simulink model "RobustStateSpaceSim"  (R2020b)
settings: Solver=ode45  StartTime=0.0  StopTime=10  RelTol=1e-3
undefined symbols (not defined in the file or in its folder): daq, degs2rpm, drv, gbox, mech, mld, mot, rads2rpm, robust, rpm2rads, sens, state_space
libraries: simulink x1
settings Model: Creator=Utente  LastModifiedBy=Utente

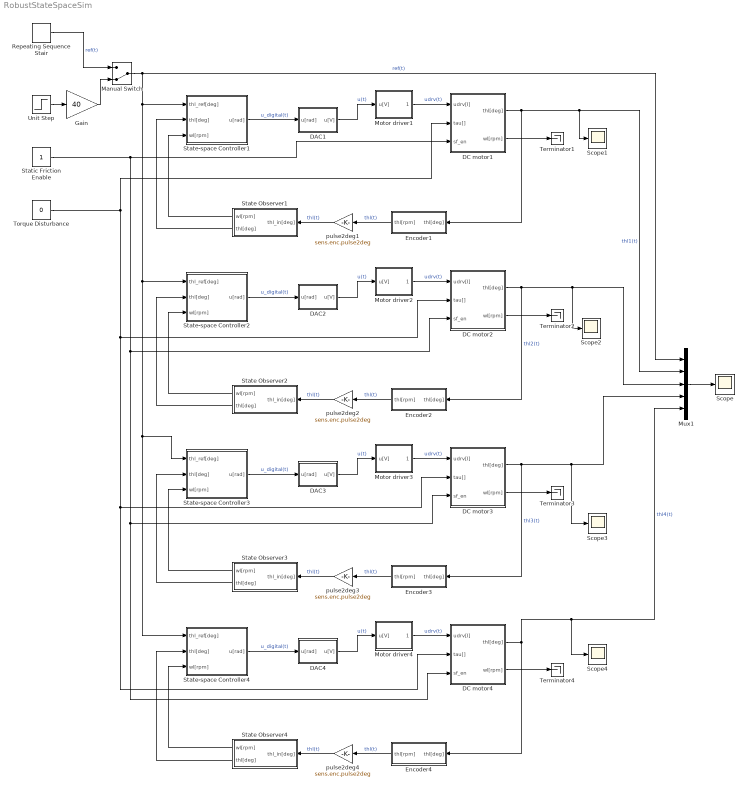
== system RobustStateSpaceSim ==
  DAC1 : Subsystem
  DAC2 : Subsystem
  DAC3 : Subsystem
  DAC4 : Subsystem
  DC motor1 : Subsystem
  DC motor2 : Subsystem
  DC motor3 : Subsystem
  DC motor4 : Subsystem
  Encoder1 : Subsystem
  Encoder2 : Subsystem
  Encoder3 : Subsystem
  Encoder4 : Subsystem
  Gain : Gain  Gain=40
  Manual Switch : ManualSwitch  CurrentSetting=0
  Motor driver1 : Subsystem
  Motor driver2 : Subsystem
  Motor driver3 : Subsystem
  Motor driver4 : Subsystem
  Mux1 : Mux  Inputs=5
  Repeating Sequence Stair : simulink/Sources/Repeating Sequence Stair  OutValues=[40 0 70 0 120 0].'  tsamp=2  OutMin=[]  OutMax=[]  OutDataTypeStr=double  OutputDataTypeScalingMode=double  OutDataType=fixdt(0,8)  ConRadixGroup=Best Precision: Vector-wise  OutScaling=2^-12
  Scope{,1..4} (5 alike) : Scope
  State Observer1 : Subsystem
  State Observer2 : Subsystem
  State Observer3 : Subsystem
  State Observer4 : Subsystem
  State-space Controller1 : Subsystem
  State-space Controller2 : Subsystem
  State-space Controller3 : Subsystem
  State-space Controller4 : Subsystem
  Static Friction Enable : Constant
  Terminator{1..4} (4 alike) : Terminator
  Torque Disturbance : Constant  Value=0
  Unit Step : Step  Time=0  SampleTime=0
  pulse2deg{1..4} (4 alike) : Gain  Gain=sens.enc.pulse2deg
  wires:
  State Observer4/2(thl[deg]) -> State-space Controller4/2(thl[deg])
  Motor driver3/1(udrv[I]) -> DC motor3/1(udrv[I])  "udrv(t)"
  State Observer4/1(wl[rpm]) -> State-space Controller4/3(wl[rpm])
  DC motor4/2(wl[rpm]) -> Terminator4/1
  DC motor3/1(thl[deg]) -> Scope3/1, Mux1/4, Encoder3/1(thl[deg])  "thl3(t)"
  DAC3/1(u[V]) -> Motor driver3/1(u[V])  "u(t)"
  State-space Controller3/1(u[rad]) -> DAC3/1(u[rad])  "u_digital(t)"
  Encoder4/1(thl[rpm]) -> pulse2deg4/1  "thl(t)"
  DC motor4/1(thl[deg]) -> Scope4/1, Mux1/5, Encoder4/1(thl[deg])  "thl4(t)"
  pulse2deg2/1 -> State Observer2/1(thl_in[deg])  "thl(t)"
  Encoder2/1(thl[rpm]) -> pulse2deg2/1  "thl(t)"
  Motor driver4/1(udrv[I]) -> DC motor4/1(udrv[I])  "udrv(t)"
  DC motor2/1(thl[deg]) -> Encoder2/1(thl[deg]), Scope2/1, Mux1/3  "thl2(t)"
  Motor driver2/1(udrv[I]) -> DC motor2/1(udrv[I])  "udrv(t)"
  DC motor3/2(wl[rpm]) -> Terminator3/1
  Manual Switch/1 -> State-space Controller3/1(thl_ref[deg]), State-space Controller4/1(thl_ref[deg]), State-space Controller2/1(thl_ref[deg]), State-space Controller1/1(thl_ref[deg]), Mux1/1  "ref(t)"
  DAC2/1(u[V]) -> Motor driver2/1(u[V])  "u(t)"
  State-space Controller2/1(u[rad]) -> DAC2/1(u[rad])  "u_digital(t)"
  State Observer1/1(wl[rpm]) -> State-space Controller1/3(wl[rpm])
  Encoder3/1(thl[rpm]) -> pulse2deg3/1  "thl(t)"
  State-space Controller1/1(u[rad]) -> DAC1/1(u[rad])  "u_digital(t)"
  pulse2deg1/1 -> State Observer1/1(thl_in[deg])  "thl(t)"
  State Observer3/1(wl[rpm]) -> State-space Controller3/3(wl[rpm])
  State Observer1/2(thl[deg]) -> State-space Controller1/2(thl[deg])
  DAC1/1(u[V]) -> Motor driver1/1(u[V])  "u(t)"
  DC motor2/2(wl[rpm]) -> Terminator2/1
  DC motor1/1(thl[deg]) -> Scope1/1, Mux1/2, Encoder1/1(thl[deg])  "thl1(t)"
  Encoder1/1(thl[rpm]) -> pulse2deg1/1  "thl(t)"
  DAC4/1(u[V]) -> Motor driver4/1(u[V])  "u(t)"
  State Observer2/1(wl[rpm]) -> State-space Controller2/3(wl[rpm])
  Motor driver1/1(udrv[I]) -> DC motor1/1(udrv[I])  "udrv(t)"
  State Observer3/2(thl[deg]) -> State-space Controller3/2(thl[deg])
  Torque Disturbance/1 -> DC motor3/2(tau[]), DC motor4/2(tau[]), DC motor2/2(tau[]), DC motor1/2(tau[])
  State-space Controller4/1(u[rad]) -> DAC4/1(u[rad])  "u_digital(t)"
  Static Friction Enable/1 -> DC motor1/3(sf_en), DC motor2/3(sf_en), DC motor3/3(sf_en), DC motor4/3(sf_en)
  pulse2deg4/1 -> State Observer4/1(thl_in[deg])  "thl(t)"
  State Observer2/2(thl[deg]) -> State-space Controller2/2(thl[deg])
  pulse2deg3/1 -> State Observer3/1(thl_in[deg])  "thl(t)"
  DC motor1/2(wl[rpm]) -> Terminator1/1
  Mux1/1 -> Scope/1
  Repeating Sequence Stair/1 -> Manual Switch/1  "ref(t)"
  Unit Step/1 -> Gain/1
  Gain/1 -> Manual Switch/2

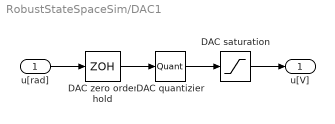
== system RobustStateSpaceSim/DAC1 ==
  u[rad] : Inport
  DAC quantizier : Quantizer  QuantizationInterval=daq.dac.q
  DAC saturation : Saturate  UpperLimit=daq.dac.vdd  LowerLimit=daq.dac.vss
  DAC zero order hold : ZeroOrderHold  SampleTime=daq.dac.T_s
  u[V] : Outport
  wires:
  DAC quantizier/1 -> DAC saturation/1
  DAC zero order hold/1 -> DAC quantizier/1
  DAC saturation/1 -> u[V]/1
  u[rad]/1 -> DAC zero order hold/1

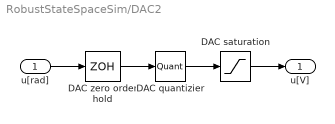
== system RobustStateSpaceSim/DAC2 ==
  u[rad] : Inport
  DAC quantizier : Quantizer  QuantizationInterval=daq.dac.q
  DAC saturation : Saturate  UpperLimit=daq.dac.vdd  LowerLimit=daq.dac.vss
  DAC zero order hold : ZeroOrderHold  SampleTime=daq.dac.T_s
  u[V] : Outport
  wires:
  DAC quantizier/1 -> DAC saturation/1
  DAC zero order hold/1 -> DAC quantizier/1
  DAC saturation/1 -> u[V]/1
  u[rad]/1 -> DAC zero order hold/1

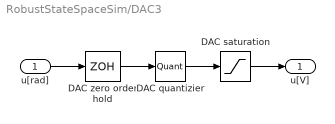
== system RobustStateSpaceSim/DAC3 ==
  u[rad] : Inport
  DAC quantizier : Quantizer  QuantizationInterval=daq.dac.q
  DAC saturation : Saturate  UpperLimit=daq.dac.vdd  LowerLimit=daq.dac.vss
  DAC zero order hold : ZeroOrderHold  SampleTime=daq.dac.T_s
  u[V] : Outport
  wires:
  DAC quantizier/1 -> DAC saturation/1
  DAC zero order hold/1 -> DAC quantizier/1
  DAC saturation/1 -> u[V]/1
  u[rad]/1 -> DAC zero order hold/1

== system RobustStateSpaceSim/DAC4 ==
  u[rad] : Inport
  DAC quantizier : Quantizer  QuantizationInterval=daq.dac.q
  DAC saturation : Saturate  UpperLimit=daq.dac.vdd  LowerLimit=daq.dac.vss
  DAC zero order hold : ZeroOrderHold  SampleTime=daq.dac.T_s
  u[V] : Outport
  wires:
  DAC quantizier/1 -> DAC saturation/1
  DAC zero order hold/1 -> DAC quantizier/1
  DAC saturation/1 -> u[V]/1
  u[rad]/1 -> DAC zero order hold/1

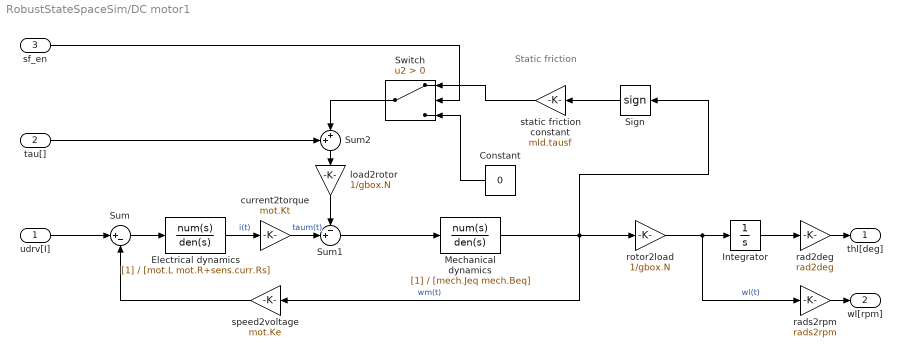
== system RobustStateSpaceSim/DC motor1 ==
  note: Static friction
  udrv[I] : Inport  Unit=V
  tau[] : Inport  Port=2  Unit=V
  sf_en : Inport  Port=3  Unit=V
  Constant : Constant  Value=0
  Electrical dynamics : TransferFcn  Denominator=[mot.L mot.R+sens.curr.Rs]
  Integrator : Integrator
  Mechanical dynamics : TransferFcn  Denominator=[mech.Jeq mech.Beq]
  Sign : Signum  ZeroCross=off
  Sum : Sum  Inputs=|+-
  Sum1 : Sum  Inputs=-+|
  Sum2 : Sum  Inputs=++|
  Switch : Switch  Criteria=u2 > Threshold
  current2torque : Gain  Gain=mot.Kt
  load2rotor : Gain  Gain=1/gbox.N
  rad2deg : Gain  Gain=rad2deg
  rads2rpm : Gain  Gain=rads2rpm
  rotor2load : Gain  Gain=1/gbox.N
  speed2voltage : Gain  Gain=mot.Ke
  static friction constant : Gain  Gain=mld.tausf
  thl[deg] : Outport  Unit=deg
  wl[rpm] : Outport  Port=2  Unit=rpm
  wires:
  load2rotor/1 -> Sum1/1
  Mechanical dynamics/1 -> Sign/1, rotor2load/1, speed2voltage/1  "wm(t)"
  Sign/1 -> static friction constant/1
  current2torque/1 -> Sum1/2  "taum(t)"
  Sum1/1 -> Mechanical dynamics/1
  speed2voltage/1 -> Sum/2
  rotor2load/1 -> rads2rpm/1, Integrator/1  "wl(t)"
  Electrical dynamics/1 -> current2torque/1  "i(t)"
  Integrator/1 -> rad2deg/1
  Sum/1 -> Electrical dynamics/1
  rads2rpm/1 -> wl[rpm]/1
  rad2deg/1 -> thl[deg]/1
  udrv[I]/1 -> Sum/1
  Sum2/1 -> load2rotor/1
  tau[]/1 -> Sum2/1
  Switch/1 -> Sum2/2
  static friction constant/1 -> Switch/1
  Constant/1 -> Switch/3
  sf_en/1 -> Switch/2

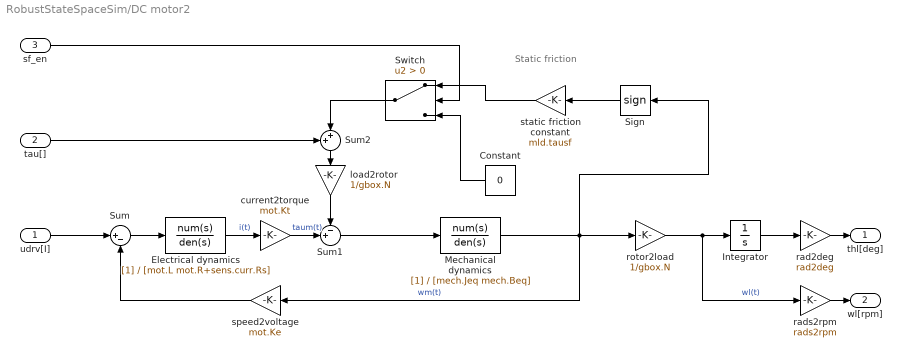
== system RobustStateSpaceSim/DC motor2 ==
  note: Static friction
  udrv[I] : Inport  Unit=V
  tau[] : Inport  Port=2  Unit=V
  sf_en : Inport  Port=3  Unit=V
  Constant : Constant  Value=0
  Electrical dynamics : TransferFcn  Denominator=[mot.L mot.R+sens.curr.Rs]
  Integrator : Integrator
  Mechanical dynamics : TransferFcn  Denominator=[mech.Jeq mech.Beq]
  Sign : Signum  ZeroCross=off
  Sum : Sum  Inputs=|+-
  Sum1 : Sum  Inputs=-+|
  Sum2 : Sum  Inputs=++|
  Switch : Switch  Criteria=u2 > Threshold
  current2torque : Gain  Gain=mot.Kt
  load2rotor : Gain  Gain=1/gbox.N
  rad2deg : Gain  Gain=rad2deg
  rads2rpm : Gain  Gain=rads2rpm
  rotor2load : Gain  Gain=1/gbox.N
  speed2voltage : Gain  Gain=mot.Ke
  static friction constant : Gain  Gain=mld.tausf
  thl[deg] : Outport  Unit=deg
  wl[rpm] : Outport  Port=2  Unit=rpm
  wires:
  load2rotor/1 -> Sum1/1
  Mechanical dynamics/1 -> Sign/1, rotor2load/1, speed2voltage/1  "wm(t)"
  Sign/1 -> static friction constant/1
  current2torque/1 -> Sum1/2  "taum(t)"
  Sum1/1 -> Mechanical dynamics/1
  speed2voltage/1 -> Sum/2
  rotor2load/1 -> rads2rpm/1, Integrator/1  "wl(t)"
  Electrical dynamics/1 -> current2torque/1  "i(t)"
  Integrator/1 -> rad2deg/1
  Sum/1 -> Electrical dynamics/1
  rads2rpm/1 -> wl[rpm]/1
  rad2deg/1 -> thl[deg]/1
  udrv[I]/1 -> Sum/1
  Sum2/1 -> load2rotor/1
  tau[]/1 -> Sum2/1
  Switch/1 -> Sum2/2
  static friction constant/1 -> Switch/1
  Constant/1 -> Switch/3
  sf_en/1 -> Switch/2

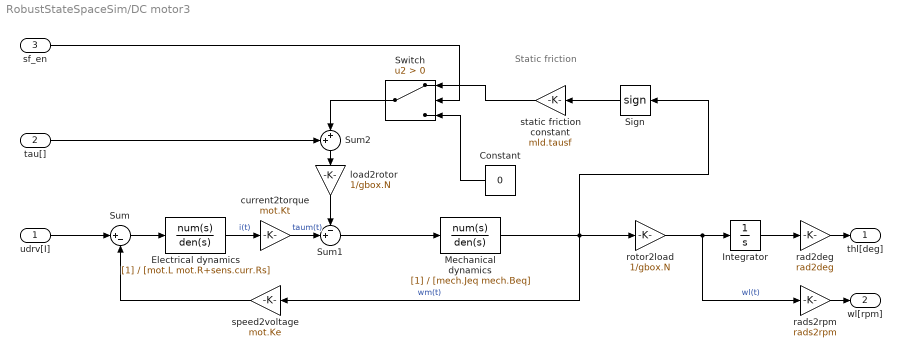
== system RobustStateSpaceSim/DC motor3 ==
  note: Static friction
  udrv[I] : Inport  Unit=V
  tau[] : Inport  Port=2  Unit=V
  sf_en : Inport  Port=3  Unit=V
  Constant : Constant  Value=0
  Electrical dynamics : TransferFcn  Denominator=[mot.L mot.R+sens.curr.Rs]
  Integrator : Integrator
  Mechanical dynamics : TransferFcn  Denominator=[mech.Jeq mech.Beq]
  Sign : Signum  ZeroCross=off
  Sum : Sum  Inputs=|+-
  Sum1 : Sum  Inputs=-+|
  Sum2 : Sum  Inputs=++|
  Switch : Switch  Criteria=u2 > Threshold
  current2torque : Gain  Gain=mot.Kt
  load2rotor : Gain  Gain=1/gbox.N
  rad2deg : Gain  Gain=rad2deg
  rads2rpm : Gain  Gain=rads2rpm
  rotor2load : Gain  Gain=1/gbox.N
  speed2voltage : Gain  Gain=mot.Ke
  static friction constant : Gain  Gain=mld.tausf
  thl[deg] : Outport  Unit=deg
  wl[rpm] : Outport  Port=2  Unit=rpm
  wires:
  load2rotor/1 -> Sum1/1
  Mechanical dynamics/1 -> Sign/1, rotor2load/1, speed2voltage/1  "wm(t)"
  Sign/1 -> static friction constant/1
  current2torque/1 -> Sum1/2  "taum(t)"
  Sum1/1 -> Mechanical dynamics/1
  speed2voltage/1 -> Sum/2
  rotor2load/1 -> rads2rpm/1, Integrator/1  "wl(t)"
  Electrical dynamics/1 -> current2torque/1  "i(t)"
  Integrator/1 -> rad2deg/1
  Sum/1 -> Electrical dynamics/1
  rads2rpm/1 -> wl[rpm]/1
  rad2deg/1 -> thl[deg]/1
  udrv[I]/1 -> Sum/1
  Sum2/1 -> load2rotor/1
  tau[]/1 -> Sum2/1
  Switch/1 -> Sum2/2
  static friction constant/1 -> Switch/1
  Constant/1 -> Switch/3
  sf_en/1 -> Switch/2

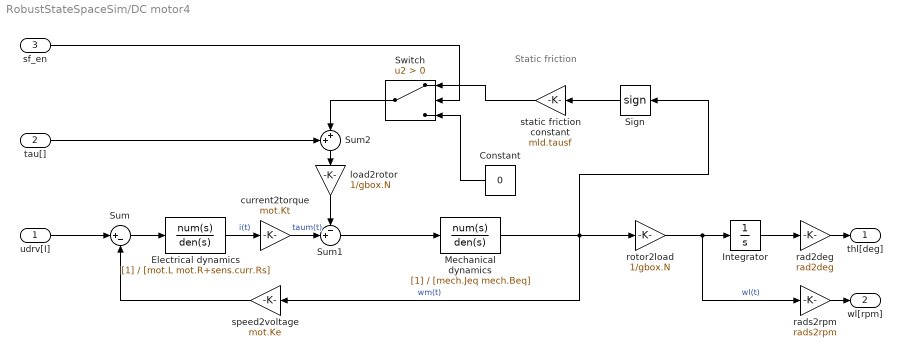
== system RobustStateSpaceSim/DC motor4 ==
  note: Static friction
  udrv[I] : Inport  Unit=V
  tau[] : Inport  Port=2  Unit=V
  sf_en : Inport  Port=3  Unit=V
  Constant : Constant  Value=0
  Electrical dynamics : TransferFcn  Denominator=[mot.L mot.R+sens.curr.Rs]
  Integrator : Integrator
  Mechanical dynamics : TransferFcn  Denominator=[mech.Jeq mech.Beq]
  Sign : Signum  ZeroCross=off
  Sum : Sum  Inputs=|+-
  Sum1 : Sum  Inputs=-+|
  Sum2 : Sum  Inputs=++|
  Switch : Switch  Criteria=u2 > Threshold
  current2torque : Gain  Gain=mot.Kt
  load2rotor : Gain  Gain=1/gbox.N
  rad2deg : Gain  Gain=rad2deg
  rads2rpm : Gain  Gain=rads2rpm
  rotor2load : Gain  Gain=1/gbox.N
  speed2voltage : Gain  Gain=mot.Ke
  static friction constant : Gain  Gain=mld.tausf
  thl[deg] : Outport  Unit=deg
  wl[rpm] : Outport  Port=2  Unit=rpm
  wires:
  load2rotor/1 -> Sum1/1
  Mechanical dynamics/1 -> Sign/1, rotor2load/1, speed2voltage/1  "wm(t)"
  Sign/1 -> static friction constant/1
  current2torque/1 -> Sum1/2  "taum(t)"
  Sum1/1 -> Mechanical dynamics/1
  speed2voltage/1 -> Sum/2
  rotor2load/1 -> rads2rpm/1, Integrator/1  "wl(t)"
  Electrical dynamics/1 -> current2torque/1  "i(t)"
  Integrator/1 -> rad2deg/1
  Sum/1 -> Electrical dynamics/1
  rads2rpm/1 -> wl[rpm]/1
  rad2deg/1 -> thl[deg]/1
  udrv[I]/1 -> Sum/1
  Sum2/1 -> load2rotor/1
  tau[]/1 -> Sum2/1
  Switch/1 -> Sum2/2
  static friction constant/1 -> Switch/1
  Constant/1 -> Switch/3
  sf_en/1 -> Switch/2

== system RobustStateSpaceSim/Encoder1 ==
  thl[deg] : Inport
  Encoder quantization : Quantizer  QuantizationInterval=sens.enc.q
  Encoder sampling : ZeroOrderHold  SampleTime=sens.enc.T_s
  deg2pulse : Gain  Gain=sens.enc.deg2pulse
  thl[rpm] : Outport
  wires:
  Encoder quantization/1 -> deg2pulse/1
  deg2pulse/1 -> thl[rpm]/1
  Encoder sampling/1 -> Encoder quantization/1
  thl[deg]/1 -> Encoder sampling/1

== system RobustStateSpaceSim/Encoder2 ==
  thl[deg] : Inport
  Encoder quantization : Quantizer  QuantizationInterval=sens.enc.q
  Encoder sampling : ZeroOrderHold  SampleTime=sens.enc.T_s
  deg2pulse : Gain  Gain=sens.enc.deg2pulse
  thl[rpm] : Outport
  wires:
  Encoder quantization/1 -> deg2pulse/1
  deg2pulse/1 -> thl[rpm]/1
  Encoder sampling/1 -> Encoder quantization/1
  thl[deg]/1 -> Encoder sampling/1

== system RobustStateSpaceSim/Encoder3 ==
  thl[deg] : Inport
  Encoder quantization : Quantizer  QuantizationInterval=sens.enc.q
  Encoder sampling : ZeroOrderHold  SampleTime=sens.enc.T_s
  deg2pulse : Gain  Gain=sens.enc.deg2pulse
  thl[rpm] : Outport
  wires:
  Encoder quantization/1 -> deg2pulse/1
  deg2pulse/1 -> thl[rpm]/1
  Encoder sampling/1 -> Encoder quantization/1
  thl[deg]/1 -> Encoder sampling/1

== system RobustStateSpaceSim/Encoder4 ==
  thl[deg] : Inport
  Encoder quantization : Quantizer  QuantizationInterval=sens.enc.q
  Encoder sampling : ZeroOrderHold  SampleTime=sens.enc.T_s
  deg2pulse : Gain  Gain=sens.enc.deg2pulse
  thl[rpm] : Outport
  wires:
  Encoder quantization/1 -> deg2pulse/1
  deg2pulse/1 -> thl[rpm]/1
  Encoder sampling/1 -> Encoder quantization/1
  thl[deg]/1 -> Encoder sampling/1

== system RobustStateSpaceSim/Motor driver1 ==
  u[V] : Inport
  Driver dynamics : TransferFcn  Numerator=[drv.dcgain]  Denominator=[drv.Tc 1]
  Driver saturation : Saturate  UpperLimit=drv.vp  LowerLimit=drv.vm
  udrv[I] : Outport
  wires:
  Driver saturation/1 -> udrv[I]/1
  Driver dynamics/1 -> Driver saturation/1
  u[V]/1 -> Driver dynamics/1

== system RobustStateSpaceSim/Motor driver2 ==
  u[V] : Inport
  Driver dynamics : TransferFcn  Numerator=[drv.dcgain]  Denominator=[drv.Tc 1]
  Driver saturation : Saturate  UpperLimit=drv.vp  LowerLimit=drv.vm
  udrv[I] : Outport
  wires:
  Driver saturation/1 -> udrv[I]/1
  Driver dynamics/1 -> Driver saturation/1
  u[V]/1 -> Driver dynamics/1

== system RobustStateSpaceSim/Motor driver3 ==
  u[V] : Inport
  Driver dynamics : TransferFcn  Numerator=[drv.dcgain]  Denominator=[drv.Tc 1]
  Driver saturation : Saturate  UpperLimit=drv.vp  LowerLimit=drv.vm
  udrv[I] : Outport
  wires:
  Driver saturation/1 -> udrv[I]/1
  Driver dynamics/1 -> Driver saturation/1
  u[V]/1 -> Driver dynamics/1

== system RobustStateSpaceSim/Motor driver4 ==
  u[V] : Inport
  Driver dynamics : TransferFcn  Numerator=[drv.dcgain]  Denominator=[drv.Tc 1]
  Driver saturation : Saturate  UpperLimit=drv.vp  LowerLimit=drv.vm
  udrv[I] : Outport
  wires:
  Driver saturation/1 -> udrv[I]/1
  Driver dynamics/1 -> Driver saturation/1
  u[V]/1 -> Driver dynamics/1

== system RobustStateSpaceSim/State Observer1 ==
  thl_in[deg] : Inport
  Gain1 : Gain  Gain=degs2rpm
  Transfer Fcn : TransferFcn  Numerator=[state_space.obs.wc^2 0]  Denominator=[1 2*state_space.obs.delta*state_space.obs.wc state_space.obs.wc^2]
  wl[rpm] : Outport
  thl[deg] : Outport  Port=2
  wires:
  Transfer Fcn/1 -> Gain1/1
  thl_in[deg]/1 -> thl[deg]/1, Transfer Fcn/1
  Gain1/1 -> wl[rpm]/1

== system RobustStateSpaceSim/State Observer2 ==
  thl_in[deg] : Inport
  Gain1 : Gain  Gain=degs2rpm
  Transfer Fcn : TransferFcn  Numerator=[state_space.obs.wc^2 0]  Denominator=[1 2*state_space.obs.delta*state_space.obs.wc state_space.obs.wc^2]
  wl[rpm] : Outport
  thl[deg] : Outport  Port=2
  wires:
  Transfer Fcn/1 -> Gain1/1
  thl_in[deg]/1 -> thl[deg]/1, Transfer Fcn/1
  Gain1/1 -> wl[rpm]/1

== system RobustStateSpaceSim/State Observer3 ==
  thl_in[deg] : Inport
  Gain1 : Gain  Gain=degs2rpm
  Transfer Fcn : TransferFcn  Numerator=[state_space.obs.wc^2 0]  Denominator=[1 2*state_space.obs.delta*state_space.obs.wc state_space.obs.wc^2]
  wl[rpm] : Outport
  thl[deg] : Outport  Port=2
  wires:
  Transfer Fcn/1 -> Gain1/1
  thl_in[deg]/1 -> thl[deg]/1, Transfer Fcn/1
  Gain1/1 -> wl[rpm]/1

== system RobustStateSpaceSim/State Observer4 ==
  thl_in[deg] : Inport
  Gain1 : Gain  Gain=degs2rpm
  Transfer Fcn : TransferFcn  Numerator=[state_space.obs.wc^2 0]  Denominator=[1 2*state_space.obs.delta*state_space.obs.wc state_space.obs.wc^2]
  wl[rpm] : Outport
  thl[deg] : Outport  Port=2
  wires:
  Transfer Fcn/1 -> Gain1/1
  thl_in[deg]/1 -> thl[deg]/1, Transfer Fcn/1
  Gain1/1 -> wl[rpm]/1

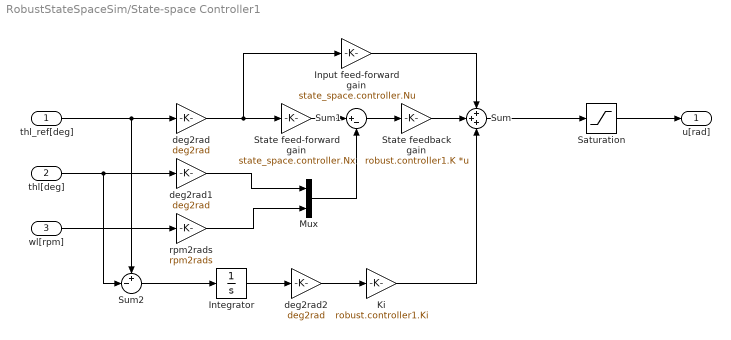
== system RobustStateSpaceSim/State-space Controller1 ==
  thl_ref[deg] : Inport
  thl[deg] : Inport  Port=2
  wl[rpm] : Inport  Port=3
  Input feed-forward gain : Gain  Gain=state_space.controller.Nu
  Integrator : Integrator
  Ki : Gain  Gain=robust.controller1.Ki
  Mux : Mux  Inputs=2
  Saturation : Saturate  UpperLimit=daq.dac.vdd  LowerLimit=daq.dac.vss
  State feed-forward gain : Gain  Gain=state_space.controller.Nx
  State feedback gain : Gain  Gain=robust.controller1.K  Multiplication=Matrix(K*u)
  Sum : Sum  Inputs=+++
  Sum1 : Sum  Inputs=|+-
  Sum2 : Sum  Inputs=+-|
  deg2rad : Gain  Gain=deg2rad
  deg2rad1 : Gain  Gain=deg2rad
  deg2rad2 : Gain  Gain=deg2rad
  rpm2rads : Gain  Gain=rpm2rads
  u[rad] : Outport
  wires:
  rpm2rads/1 -> Mux/2
  Sum1/1 -> State feedback gain/1
  Mux/1 -> Sum1/2
  thl_ref[deg]/1 -> Sum2/1, deg2rad/1
  deg2rad/1 -> Input feed-forward gain/1, State feed-forward gain/1
  State feed-forward gain/1 -> Sum1/1
  deg2rad1/1 -> Mux/1
  Input feed-forward gain/1 -> Sum/1
  Saturation/1 -> u[rad]/1
  wl[rpm]/1 -> rpm2rads/1
  thl[deg]/1 -> Sum2/2, deg2rad1/1
  State feedback gain/1 -> Sum/2
  Sum/1 -> Saturation/1
  Sum2/1 -> Integrator/1
  Integrator/1 -> deg2rad2/1
  deg2rad2/1 -> Ki/1
  Ki/1 -> Sum/3

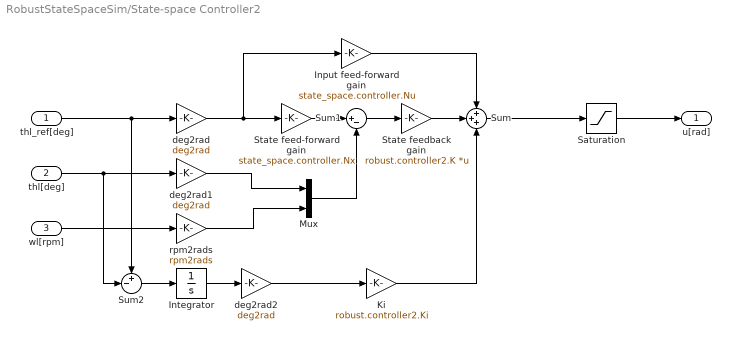
== system RobustStateSpaceSim/State-space Controller2 ==
  thl_ref[deg] : Inport
  thl[deg] : Inport  Port=2
  wl[rpm] : Inport  Port=3
  Input feed-forward gain : Gain  Gain=state_space.controller.Nu
  Integrator : Integrator
  Ki : Gain  Gain=robust.controller2.Ki
  Mux : Mux  Inputs=2
  Saturation : Saturate  UpperLimit=daq.dac.vdd  LowerLimit=daq.dac.vss
  State feed-forward gain : Gain  Gain=state_space.controller.Nx
  State feedback gain : Gain  Gain=robust.controller2.K  Multiplication=Matrix(K*u)
  Sum : Sum  Inputs=+++
  Sum1 : Sum  Inputs=|+-
  Sum2 : Sum  Inputs=+-|
  deg2rad : Gain  Gain=deg2rad
  deg2rad1 : Gain  Gain=deg2rad
  deg2rad2 : Gain  Gain=deg2rad
  rpm2rads : Gain  Gain=rpm2rads
  u[rad] : Outport
  wires:
  rpm2rads/1 -> Mux/2
  Sum1/1 -> State feedback gain/1
  Mux/1 -> Sum1/2
  thl_ref[deg]/1 -> Sum2/1, deg2rad/1
  deg2rad/1 -> Input feed-forward gain/1, State feed-forward gain/1
  State feed-forward gain/1 -> Sum1/1
  deg2rad1/1 -> Mux/1
  Input feed-forward gain/1 -> Sum/1
  Saturation/1 -> u[rad]/1
  wl[rpm]/1 -> rpm2rads/1
  thl[deg]/1 -> Sum2/2, deg2rad1/1
  State feedback gain/1 -> Sum/2
  Sum/1 -> Saturation/1
  Sum2/1 -> Integrator/1
  Integrator/1 -> deg2rad2/1
  deg2rad2/1 -> Ki/1
  Ki/1 -> Sum/3

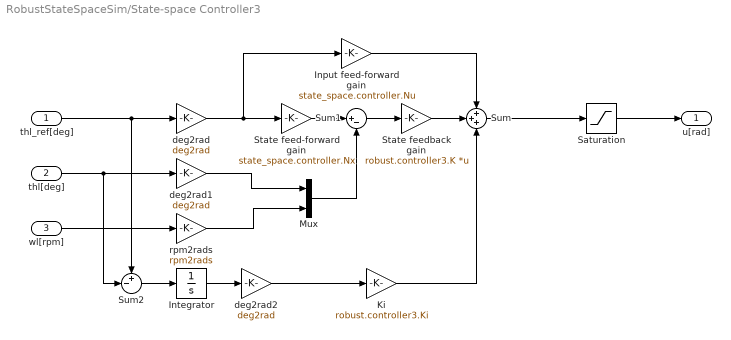
== system RobustStateSpaceSim/State-space Controller3 ==
  thl_ref[deg] : Inport
  thl[deg] : Inport  Port=2
  wl[rpm] : Inport  Port=3
  Input feed-forward gain : Gain  Gain=state_space.controller.Nu
  Integrator : Integrator
  Ki : Gain  Gain=robust.controller3.Ki
  Mux : Mux  Inputs=2
  Saturation : Saturate  UpperLimit=daq.dac.vdd  LowerLimit=daq.dac.vss
  State feed-forward gain : Gain  Gain=state_space.controller.Nx
  State feedback gain : Gain  Gain=robust.controller3.K  Multiplication=Matrix(K*u)
  Sum : Sum  Inputs=+++
  Sum1 : Sum  Inputs=|+-
  Sum2 : Sum  Inputs=+-|
  deg2rad : Gain  Gain=deg2rad
  deg2rad1 : Gain  Gain=deg2rad
  deg2rad2 : Gain  Gain=deg2rad
  rpm2rads : Gain  Gain=rpm2rads
  u[rad] : Outport
  wires:
  rpm2rads/1 -> Mux/2
  Sum1/1 -> State feedback gain/1
  Mux/1 -> Sum1/2
  thl_ref[deg]/1 -> Sum2/1, deg2rad/1
  deg2rad/1 -> Input feed-forward gain/1, State feed-forward gain/1
  State feed-forward gain/1 -> Sum1/1
  deg2rad1/1 -> Mux/1
  Input feed-forward gain/1 -> Sum/1
  Saturation/1 -> u[rad]/1
  wl[rpm]/1 -> rpm2rads/1
  thl[deg]/1 -> Sum2/2, deg2rad1/1
  State feedback gain/1 -> Sum/2
  Sum/1 -> Saturation/1
  Sum2/1 -> Integrator/1
  Integrator/1 -> deg2rad2/1
  deg2rad2/1 -> Ki/1
  Ki/1 -> Sum/3

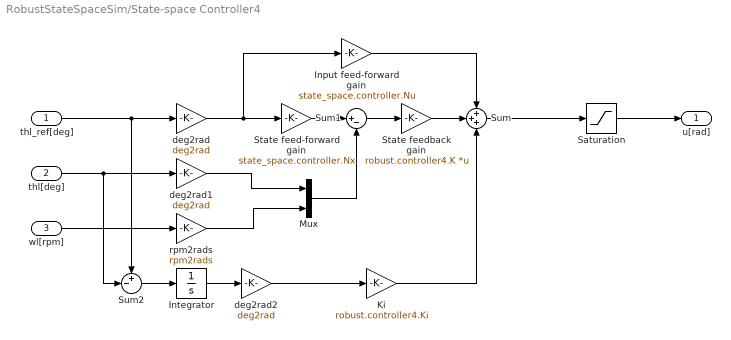
== system RobustStateSpaceSim/State-space Controller4 ==
  thl_ref[deg] : Inport
  thl[deg] : Inport  Port=2
  wl[rpm] : Inport  Port=3
  Input feed-forward gain : Gain  Gain=state_space.controller.Nu
  Integrator : Integrator
  Ki : Gain  Gain=robust.controller4.Ki
  Mux : Mux  Inputs=2
  Saturation : Saturate  UpperLimit=daq.dac.vdd  LowerLimit=daq.dac.vss
  State feed-forward gain : Gain  Gain=state_space.controller.Nx
  State feedback gain : Gain  Gain=robust.controller4.K  Multiplication=Matrix(K*u)
  Sum : Sum  Inputs=+++
  Sum1 : Sum  Inputs=|+-
  Sum2 : Sum  Inputs=+-|
  deg2rad : Gain  Gain=deg2rad
  deg2rad1 : Gain  Gain=deg2rad
  deg2rad2 : Gain  Gain=deg2rad
  rpm2rads : Gain  Gain=rpm2rads
  u[rad] : Outport
  wires:
  rpm2rads/1 -> Mux/2
  Sum1/1 -> State feedback gain/1
  Mux/1 -> Sum1/2
  thl_ref[deg]/1 -> Sum2/1, deg2rad/1
  deg2rad/1 -> Input feed-forward gain/1, State feed-forward gain/1
  State feed-forward gain/1 -> Sum1/1
  deg2rad1/1 -> Mux/1
  Input feed-forward gain/1 -> Sum/1
  Saturation/1 -> u[rad]/1
  wl[rpm]/1 -> rpm2rads/1
  thl[deg]/1 -> Sum2/2, deg2rad1/1
  State feedback gain/1 -> Sum/2
  Sum/1 -> Saturation/1
  Sum2/1 -> Integrator/1
  Integrator/1 -> deg2rad2/1
  deg2rad2/1 -> Ki/1
  Ki/1 -> Sum/3
